simulink model "MA_filter_sim_types"  (R2020b)
settings: Solver=FixedStepAuto  StartTime=0.0  StopTime=10.0  FixedStep=Ts  RelTol=1e-3
values from neighbouring files (symbols this model uses):
  N = T_MAF/Ts    (= 200)    [maf_filter.m]
  Ts = 1/fs    (= 0.0001)    [maf_filter.m]
undefined symbols (not defined in the file or in its folder): f_rad
libraries: dspstat3 x14, dspsrcs4 x4
settings Model: Creator=Kasper Laustsen  LastModifiedBy=Kasper Laustsen

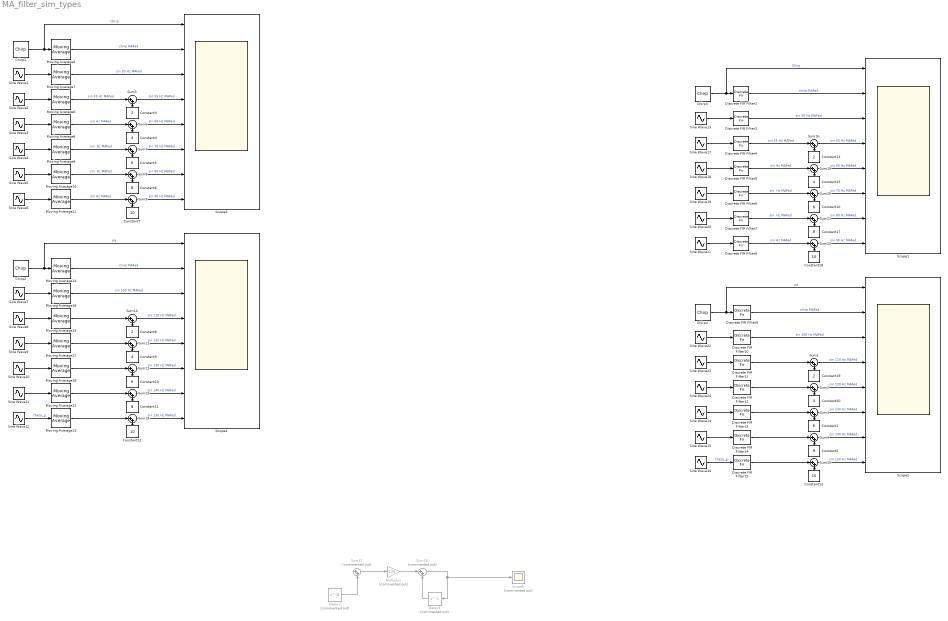
== system MA_filter_sim_types ==
  Chirp1 : dspsrcs4/Chirp  sweep=Linear  mode=Unidirectional  f0=0  f1=100  t1=2  Tsweep=2  phase=0  Ts=Ts  spf=1  datatype=Double  OutputFrames=off
  Chirp2 : dspsrcs4/Chirp  sweep=Linear  mode=Bidirectional  f0=0  f1=100  t1=2  Tsweep=2  phase=0  Ts=Ts  spf=1  datatype=Double  OutputFrames=off
  Chirp3 : dspsrcs4/Chirp  sweep=Linear  mode=Unidirectional  f0=0  f1=100  t1=2  Tsweep=2  phase=0  Ts=Ts  spf=1  datatype=Double  OutputFrames=off
  Chirp4 : dspsrcs4/Chirp  sweep=Linear  mode=Bidirectional  f0=0  f1=100  t1=2  Tsweep=2  phase=0  Ts=Ts  spf=1  datatype=Double  OutputFrames=off
  Constant{1,5,10,16} (4 alike) : Constant  Value=6
  Constant{2,6,11,17} (4 alike) : Constant  Value=8
  Constant{7,12..13,18} (4 alike) : Constant  Value=10
  Constant{3,8,14,19} (4 alike) : Constant  Value=2
  Constant{4,9,15,20} (4 alike) : Constant  Value=4
  Delay2 : Delay  Commented=on  DelayLength=N  SampleTime=Ts
  Delay3 : Delay  Commented=on  DelayLength=1  SampleTime=Ts
  Discrete FIR Filter{1..2,4..15} (14 alike) : DiscreteFir  Coefficients=[ones(1,N).*1/N]
  Moving Average{5..18} (14 alike) : dspstat3/Moving Average  Method=Sliding window  ForgettingFactorPort=off  SpecifyWindowLength=on  WindowLength=N  ForgettingFactor=0.9  SimulateUsing=Code generation
  Multiply1 : Gain  Commented=on  Gain=1/N
  Scope{1..4} (4 alike) : Scope  NumInputPorts=8
  Scope6 : Scope  Commented=on
  Sine Wave1 : Sin  Frequency=f_rad  Phase=pi/2  SampleTime=0
  Sine Wave10 : Sin  Frequency=f_rad*2.6  Phase=pi/2  SampleTime=0
  Sine Wave11 : Sin  Frequency=f_rad*2.8  Phase=pi/2  SampleTime=0
  Sine Wave12 : Sin  Frequency=f_rad*3  Phase=pi/2  SampleTime=0
  Sine Wave13 : Sin  Frequency=f_rad  Phase=pi/2  SampleTime=0
  Sine Wave14 : Sin  Frequency=f_rad*2.6  Phase=pi/2  SampleTime=0
  Sine Wave15 : Sin  Frequency=f_rad*2.8  Phase=pi/2  SampleTime=0
  Sine Wave16 : Sin  Frequency=f_rad*3  Phase=pi/2  SampleTime=0
  Sine Wave17 : Sin  Frequency=f_rad*1.1  Phase=pi/2  SampleTime=0
  Sine Wave18 : Sin  Frequency=f_rad*1.2  Phase=pi/2  SampleTime=0
  Sine Wave19 : Sin  Frequency=f_rad*1.4  Phase=pi/2  SampleTime=0
  Sine Wave2 : Sin  Frequency=f_rad*1.1  Phase=pi/2  SampleTime=0
  Sine Wave20 : Sin  Frequency=f_rad*1.6  Phase=pi/2  SampleTime=0
  Sine Wave21 : Sin  Frequency=f_rad*1.8  Phase=pi/2  SampleTime=0
  Sine Wave22 : Sin  Frequency=f_rad*2  Phase=pi/2  SampleTime=0
  Sine Wave23 : Sin  Frequency=f_rad*2.2  Phase=pi/2  SampleTime=0
  Sine Wave24 : Sin  Frequency=f_rad*2.4  Phase=pi/2  SampleTime=0
  Sine Wave3 : Sin  Frequency=f_rad*1.2  Phase=pi/2  SampleTime=0
  Sine Wave4 : Sin  Frequency=f_rad*1.4  Phase=pi/2  SampleTime=0
  Sine Wave5 : Sin  Frequency=f_rad*1.6  Phase=pi/2  SampleTime=0
  Sine Wave6 : Sin  Frequency=f_rad*1.8  Phase=pi/2  SampleTime=0
  Sine Wave7 : Sin  Frequency=f_rad*2  Phase=pi/2  SampleTime=0
  Sine Wave8 : Sin  Frequency=f_rad*2.2  Phase=pi/2  SampleTime=0
  Sine Wave9 : Sin  Frequency=f_rad*2.4  Phase=pi/2  SampleTime=0
  Sum{1..16,19..22} (20 alike) : Sum  Inputs=|++
  Sum17 : Sum  Commented=on  Inputs=|++
  Sum18 : Sum  Commented=on  Inputs=|++
  wires:
  Constant6/1 -> Sum8/2
  Sine Wave4/1 -> Moving Average9/1
  Moving Average9/1 -> Sum7/1  "sin  Hz MAFed"
  Constant3/1 -> Sum5/2
  Sine Wave3/1 -> Moving Average8/1
  Sine Wave6/1 -> Moving Average11/1
  Moving Average11/1 -> Sum9/1  "sin Hz MAFed"
  Moving Average8/1 -> Sum6/1  "sin Hz MAFed"
  Constant7/1 -> Sum9/2
  Sine Wave2/1 -> Moving Average6/1
  Moving Average7/1 -> Scope3/3  "sin 50 Hz MAFed"
  Constant5/1 -> Sum7/2
  Sum8/1 -> Scope3/7  "sin 80 Hz MAFed"
  Sum5/1 -> Scope3/4  "sin 55 Hz MAFed"
  Constant9/1 -> Sum11/2
  Sum6/1 -> Scope3/5  "sin 60 Hz MAFed"
  Chirp2/1 -> Scope4/1, Moving Average14/1  "pa"
  Sine Wave11/1 -> Moving Average12/1
  Sine Wave7/1 -> Moving Average16/1
  Moving Average10/1 -> Sum8/1  "sin  Hz MAFed"
  Moving Average17/1 -> Sum11/1
  Moving Average13/1 -> Sum14/1
  Moving Average15/1 -> Sum10/1
  Moving Average12/1 -> Sum13/1
  Sine Wave10/1 -> Moving Average18/1
  Moving Average18/1 -> Sum12/1
  Constant8/1 -> Sum10/2
  Sine Wave12/1 -> Moving Average13/1  "theta_g"
  Constant11/1 -> Sum13/2
  Moving Average6/1 -> Sum5/1  "sin 55 Hz MAFed"
  Moving Average14/1 -> Scope4/2  "chirp MAFed"
  Sum14/1 -> Scope4/8  "sin 150 Hz MAFed"
  Sine Wave8/1 -> Moving Average15/1
  Sum13/1 -> Scope4/7  "sin 140 Hz MAFed"
  Sum11/1 -> Scope4/5  "sin 120 Hz MAFed"
  Constant12/1 -> Sum14/2
  Sum10/1 -> Scope4/4  "sin 110 Hz MAFed"
  Sum9/1 -> Scope3/8  "sin 90 Hz MAFed"
  Sum12/1 -> Scope4/6  "sin 130 Hz MAFed"
  Moving Average5/1 -> Scope3/2  "chirp MAFed"
  Sine Wave9/1 -> Moving Average17/1
  Constant10/1 -> Sum12/2
  Sum7/1 -> Scope3/6  "sin 70 Hz MAFed"
  Sine Wave1/1 -> Moving Average7/1
  Moving Average16/1 -> Scope4/3  "sin 100 Hz MAFed"
  Chirp1/1 -> Scope3/1, Moving Average5/1  "Chirp"
  Sine Wave5/1 -> Moving Average10/1
  Constant4/1 -> Sum6/2
  ? -> Sum17/1, Delay2/1  "theta_g"
  Sum18/1 -> Delay3/1, Scope6/1
  Delay2/1 -> Sum17/2
  Delay3/1 -> Sum18/2
  Multiply1/1 -> Sum18/1
  Sum17/1 -> Multiply1/1
  Constant1/1 -> Sum3/2
  Sum20/1 -> Scope1/6  "sin 70 Hz MAFed"
  Constant13/1 -> Sum15/2
  Sum3/1 -> Scope2/6  "sin 130 Hz MAFed"
  Discrete FIR Filter1/1 -> Scope1/2  "chirp MAFed"
  Sum1/1 -> Scope2/4  "sin 110 Hz MAFed"
  Sum22/1 -> Scope1/8  "sin 90 Hz MAFed"
  Constant15/1 -> Sum19/2
  Discrete FIR Filter10/1 -> Scope2/3  "sin 100 Hz MAFed"
  Sine Wave13/1 -> Discrete FIR Filter2/1
  Chirp3/1 -> Discrete FIR Filter1/1, Scope1/1  "Chirp"
  Sine Wave16/1 -> Discrete FIR Filter15/1  "theta_g"
  Discrete FIR Filter9/1 -> Scope2/2  "chirp MAFed"
  Discrete FIR Filter15/1 -> Sum15/1
  Sine Wave14/1 -> Discrete FIR Filter13/1
  Discrete FIR Filter13/1 -> Sum3/1
  Discrete FIR Filter12/1 -> Sum2/1
  Constant19/1 -> Sum1/2
  Sine Wave20/1 -> Discrete FIR Filter7/1
  Chirp4/1 -> Discrete FIR Filter9/1, Scope2/1  "pa"
  Sine Wave15/1 -> Discrete FIR Filter14/1
  Sine Wave24/1 -> Discrete FIR Filter12/1
  Sum19/1 -> Scope1/5  "sin 60 Hz MAFed"
  Discrete FIR Filter14/1 -> Sum4/1
  Discrete FIR Filter5/1 -> Sum19/1  "sin Hz MAFed"
  Constant18/1 -> Sum22/2
  Sine Wave17/1 -> Discrete FIR Filter4/1
  Constant20/1 -> Sum2/2
  Sum16/1 -> Scope1/4  "sin 55 Hz MAFed"
  Sum21/1 -> Scope1/7  "sin 80 Hz MAFed"
  Sum15/1 -> Scope2/8  "sin 150 Hz MAFed"
  Discrete FIR Filter4/1 -> Sum16/1  "sin 55 Hz MAFed"
  Constant16/1 -> Sum20/2
  Constant14/1 -> Sum16/2
  Constant17/1 -> Sum21/2
  Sine Wave21/1 -> Discrete FIR Filter8/1
  Discrete FIR Filter6/1 -> Sum20/1  "sin  Hz MAFed"
  Sum2/1 -> Scope2/5  "sin 120 Hz MAFed"
  Discrete FIR Filter2/1 -> Scope1/3  "sin 50 Hz MAFed"
  Discrete FIR Filter11/1 -> Sum1/1
  Discrete FIR Filter8/1 -> Sum22/1  "sin Hz MAFed"
  Discrete FIR Filter7/1 -> Sum21/1  "sin  Hz MAFed"
  Constant2/1 -> Sum4/2
  Sine Wave19/1 -> Discrete FIR Filter6/1
  Sum4/1 -> Scope2/7  "sin 140 Hz MAFed"
  Sine Wave23/1 -> Discrete FIR Filter11/1
  Sine Wave18/1 -> Discrete FIR Filter5/1
  Sine Wave22/1 -> Discrete FIR Filter10/1
